simulink model "hw2_2_simu"  (R2015a)
settings: Solver=ode45  StartTime=0.0  StopTime=50  FixedStep=0.5  RelTol=1e-3
settings Model: Creator=DELL-  LastModifiedBy=DELL-

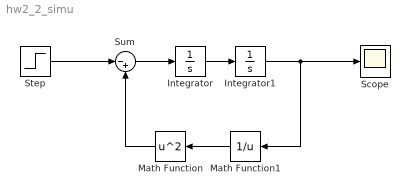
== system hw2_2_simu ==
  Integrator : Integrator
  Integrator1 : Integrator  InitialCondition=0.2
  Math Function : Math  Operator=square  SaturateOnIntegerOverflow=on
  Math Function1 : Math  Operator=reciprocal  SaturateOnIntegerOverflow=on
  Scope : Scope
  Step : Step  SampleTime=0
  Sum : Sum  Inputs=|-+
  wires:
  Step/1 -> Sum/1
  Sum/1 -> Integrator/1
  Integrator/1 -> Integrator1/1
  Integrator1/1 -> Math Function1/1, Scope/1
  Math Function1/1 -> Math Function/1
  Math Function/1 -> Sum/2
